simulink model "BCM_C1A_CombiSwitch_9"  (Simulink 9.2)
settings: Solver=FixedStepDiscrete  StartTime=0.0  StopTime=10.0  FixedStep=0.01  RelTol=1e-3
undefined symbols (not defined in the file or in its folder): TYP_VEHICLE_STATE
libraries: Renault_Library x8, library_BCM x1
settings Model: Creator=a205328  LastModifiedBy=40005501
settings DataIOCC: SaveFormat=StructureWithTime
settings OptimizationCC: ExpressionDepthLimit=2147483647
settings DebuggingCC: SolverPrmCheckMsg=warning  InheritedTsInSrcMsg=none
settings HardwareCC: TargetBitPerPointer=64  TargetBitPerSizeT=64  TargetBitPerPtrDiffT=64  TargetLongLongMode=on  TargetIntDivRoundTo=Zero  TargetEndianess=LittleEndian  TargetWordSize=64  TargetHWDeviceType=MATLAB Host  ProdEqTarget=off
settings GRTTargetCC: MatFileLogging=off  SupportNonFinite=off
settings ConfigComp: CovMetricSettings=dcmw  CovHTMLOptions=-sRT=1 -aTS=1 -bRG=1 -bTC=1 -hTR=0 -nFC=0 -scm=1 -bcm=1 -xEv=0  DVMaxTestCaseSteps=500  DVTestSuiteOptimization=CombinedObjectives (Nonlinear Extended)  DVDetectDeadLogic=on  DVDetectActiveLogic=on  DVDetectDivisionByZero=off  DVDetectIntegerOverflow=off

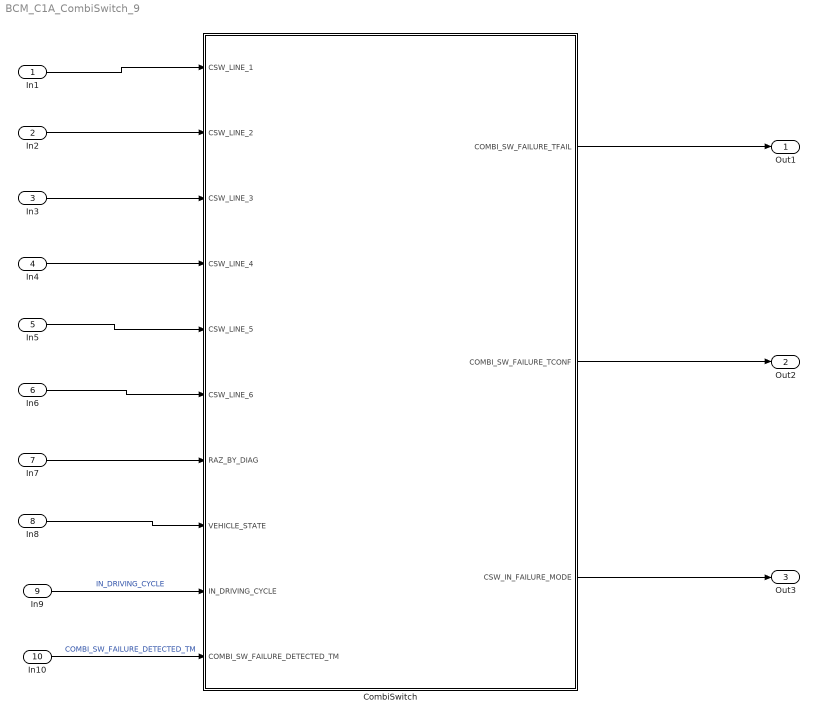
== system BCM_C1A_CombiSwitch_9 ==
  In1 : Inport
  In2 : Inport  Port=2
  In3 : Inport  Port=3
  In4 : Inport  Port=4
  In5 : Inport  Port=5
  In6 : Inport  Port=6
  In7 : Inport  Port=7
  In8 : Inport  Port=8
  In9 : Inport  Port=9
  In10 : Inport  Port=10
  CombiSwitch : Subsystem  Tag=[RUNNABLE]
  Out1 : Outport
  Out2 : Outport  Port=2
  Out3 : Outport  Port=3
  wires:
  In2/1 -> CombiSwitch/2(CSW_LINE_2)
  In3/1 -> CombiSwitch/3(CSW_LINE_3)
  In4/1 -> CombiSwitch/4(CSW_LINE_4)
  In7/1 -> CombiSwitch/7(RAZ_BY_DIAG)
  In1/1 -> CombiSwitch/1(CSW_LINE_1)
  In5/1 -> CombiSwitch/5(CSW_LINE_5)
  In6/1 -> CombiSwitch/6(CSW_LINE_6)
  In8/1 -> CombiSwitch/8(VEHICLE_STATE)
  CombiSwitch/1(COMBI_SW_FAILURE_TFAIL) -> Out1/1
  CombiSwitch/2(COMBI_SW_FAILURE_TCONF) -> Out2/1
  CombiSwitch/3(CSW_IN_FAILURE_MODE) -> Out3/1
  In9/1 -> CombiSwitch/9(IN_DRIVING_CYCLE)  "IN_DRIVING_CYCLE"
  In10/1 -> CombiSwitch/10(COMBI_SW_FAILURE_DETECTED_TM)  "COMBI_SW_FAILURE_DETECTED_TM"

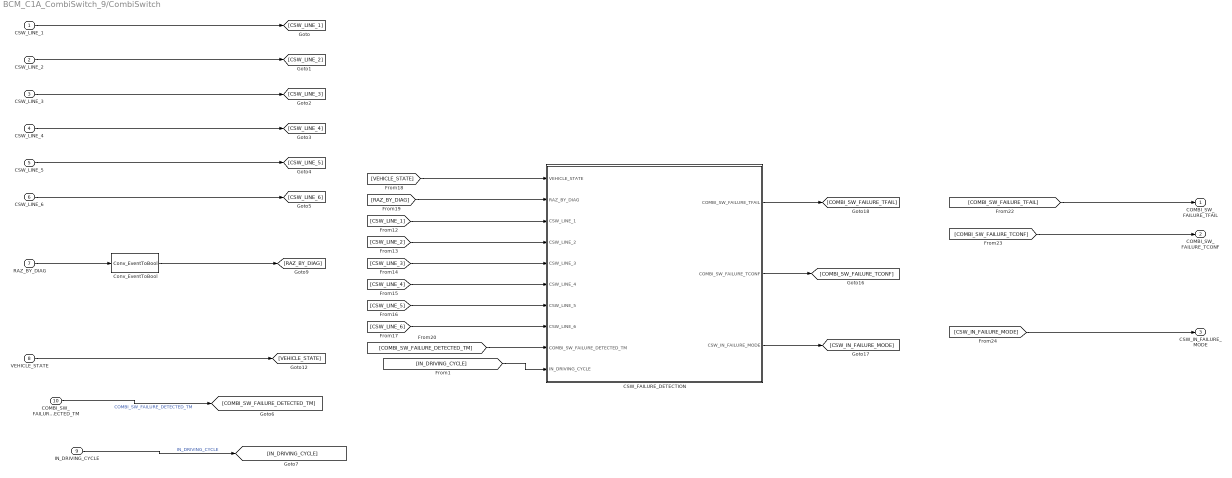
== system BCM_C1A_CombiSwitch_9/CombiSwitch ==
  CSW_LINE_1 : Inport  OutDataTypeStr=boolean  PortDimensions=6
      settings: AttributesFormatString=Type : %<OutDataTypeStr>
  CSW_LINE_2 : Inport  Port=2  OutDataTypeStr=boolean  PortDimensions=6
      settings: AttributesFormatString=Type : %<OutDataTypeStr>
  CSW_LINE_3 : Inport  Port=3  OutDataTypeStr=boolean  PortDimensions=6
      settings: AttributesFormatString=Type : %<OutDataTypeStr>
  CSW_LINE_4 : Inport  Port=4  OutDataTypeStr=boolean  PortDimensions=6
      settings: AttributesFormatString=Type : %<OutDataTypeStr>
  CSW_LINE_5 : Inport  Port=5  OutDataTypeStr=boolean  PortDimensions=6
      settings: AttributesFormatString=Type : %<OutDataTypeStr>
  CSW_LINE_6 : Inport  Port=6  OutDataTypeStr=boolean  PortDimensions=6
      settings: AttributesFormatString=Type : %<OutDataTypeStr>
  RAZ_BY_DIAG : Inport  Port=7  OutDataTypeStr=Enum: TYP_EVENT
      settings: AttributesFormatString=Type : %<OutDataTypeStr>
  VEHICLE_STATE : Inport  Port=8  OutDataTypeStr=Enum: TYP_VEHICLE_STATE
      settings: AttributesFormatString=Type : %<OutDataTypeStr>
  IN_DRIVING_CYCLE : Inport  Port=9  OutDataTypeStr=boolean
      settings: AttributesFormatString=Type : %<OutDataTypeStr>
  COMBI_SW_FAILURE_DETECTED_TM : Inport  Port=10  OutDataTypeStr=uint16
      settings: AttributesFormatString=Type : %<OutDataTypeStr>
  CSW_FAILURE_DETECTION : Subsystem  Description=|
      | RQT_BCM_CSV_1_1  
      | RQT_BCM_CSV_1_2  
      | RQT_BCM_CSV_1_3  
      | RQT_BCM_CSV_1_3_2
  Conv_EventToBool : library_BCM/Modeling/Conv_EventToBool
  COMBI_SW_FAILURE_TFAIL : Outport  OutDataTypeStr=boolean
      settings: AttributesFormatString=Type : %<OutDataTypeStr>\nInit :%<InitialOutput>
  COMBI_SW_FAILURE_TCONF : Outport  Port=2  OutDataTypeStr=boolean
      settings: AttributesFormatString=Type : %<OutDataTypeStr>\nInit :%<InitialOutput>
  CSW_IN_FAILURE_MODE : Outport  Port=3  OutDataTypeStr=boolean
      settings: AttributesFormatString=Type : %<OutDataTypeStr>\nInit :%<InitialOutput>
  wires:
  Conv_EventToBool/1 -> [RAZ_BY_DIAG]
  [COMBI_SW_FAILURE_DETECTED_TM] -> CSW_FAILURE_DETECTION/9(COMBI_SW_FAILURE_DETECTED_TM)
  [CSW_LINE_6] -> CSW_FAILURE_DETECTION/8(CSW_LINE_6)
  [CSW_LINE_5] -> CSW_FAILURE_DETECTION/7(CSW_LINE_5)
  [CSW_LINE_4] -> CSW_FAILURE_DETECTION/6(CSW_LINE_4)
  [CSW_LINE_3] -> CSW_FAILURE_DETECTION/5(CSW_LINE_3)
  [CSW_LINE_2] -> CSW_FAILURE_DETECTION/4(CSW_LINE_2)
  [CSW_LINE_1] -> CSW_FAILURE_DETECTION/3(CSW_LINE_1)
  [RAZ_BY_DIAG] -> CSW_FAILURE_DETECTION/2(RAZ_BY_DIAG)
  [VEHICLE_STATE] -> CSW_FAILURE_DETECTION/1(VEHICLE_STATE)
  CSW_LINE_6/1 -> [CSW_LINE_6]
  CSW_LINE_5/1 -> [CSW_LINE_5]
  CSW_LINE_4/1 -> [CSW_LINE_4]
  CSW_LINE_3/1 -> [CSW_LINE_3]
  CSW_LINE_2/1 -> [CSW_LINE_2]
  CSW_LINE_1/1 -> [CSW_LINE_1]
  RAZ_BY_DIAG/1 -> Conv_EventToBool/1
  VEHICLE_STATE/1 -> [VEHICLE_STATE]
  CSW_FAILURE_DETECTION/2(COMBI_SW_FAILURE_TCONF) -> [COMBI_SW_FAILURE_TCONF]
  CSW_FAILURE_DETECTION/3(CSW_IN_FAILURE_MODE) -> [CSW_IN_FAILURE_MODE]
  CSW_FAILURE_DETECTION/1(COMBI_SW_FAILURE_TFAIL) -> [COMBI_SW_FAILURE_TFAIL]
  [COMBI_SW_FAILURE_TFAIL] -> COMBI_SW_FAILURE_TFAIL/1
  [COMBI_SW_FAILURE_TCONF] -> COMBI_SW_FAILURE_TCONF/1
  [CSW_IN_FAILURE_MODE] -> CSW_IN_FAILURE_MODE/1
  [IN_DRIVING_CYCLE] -> CSW_FAILURE_DETECTION/10(IN_DRIVING_CYCLE)
  IN_DRIVING_CYCLE/1 -> [IN_DRIVING_CYCLE]  "IN_DRIVING_CYCLE"
  COMBI_SW_FAILURE_DETECTED_TM/1 -> [COMBI_SW_FAILURE_DETECTED_TM]  "COMBI_SW_FAILURE_DETECTED_TM"

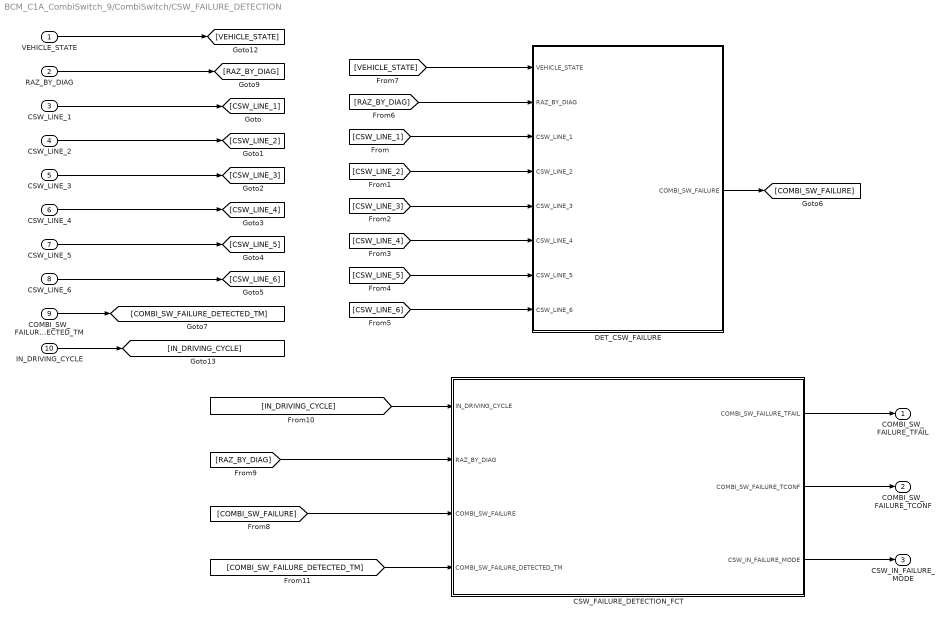
== system BCM_C1A_CombiSwitch_9/CombiSwitch/CSW_FAILURE_DETECTION ==
  VEHICLE_STATE : Inport  OutDataTypeStr=Enum: TYP_VEHICLE_STATE
      settings: AttributesFormatString=Type : %<OutDataTypeStr>
  RAZ_BY_DIAG : Inport  Port=2  OutDataTypeStr=boolean
      settings: AttributesFormatString=Type : %<OutDataTypeStr>
  CSW_LINE_1 : Inport  Port=3  OutDataTypeStr=boolean  PortDimensions=6
      settings: AttributesFormatString=Type : %<OutDataTypeStr>
  CSW_LINE_2 : Inport  Port=4  OutDataTypeStr=boolean  PortDimensions=6
      settings: AttributesFormatString=Type : %<OutDataTypeStr>
  CSW_LINE_3 : Inport  Port=5  OutDataTypeStr=boolean  PortDimensions=6
      settings: AttributesFormatString=Type : %<OutDataTypeStr>
  CSW_LINE_4 : Inport  Port=6  OutDataTypeStr=boolean  PortDimensions=6
      settings: AttributesFormatString=Type : %<OutDataTypeStr>
  CSW_LINE_5 : Inport  Port=7  OutDataTypeStr=boolean  PortDimensions=6
      settings: AttributesFormatString=Type : %<OutDataTypeStr>
  CSW_LINE_6 : Inport  Port=8  OutDataTypeStr=boolean  PortDimensions=6
      settings: AttributesFormatString=Type : %<OutDataTypeStr>
  COMBI_SW_FAILURE_DETECTED_TM : Inport  Port=9  OutDataTypeStr=uint16
      settings: AttributesFormatString=Type : %<OutDataTypeStr>
  IN_DRIVING_CYCLE : Inport  Port=10  OutDataTypeStr=boolean
      settings: AttributesFormatString=Type : %<OutDataTypeStr>
  CSW_FAILURE_DETECTION_FCT : Stateflow chart  Description=RQT_BCM_CSV_1_0_1  TreatAsAtomicUnit=on
  DET_CSW_FAILURE : Subsystem
  COMBI_SW_FAILURE_TFAIL : Outport  OutDataTypeStr=boolean
      settings: AttributesFormatString=Type : %<OutDataTypeStr>\nInit :%<InitialOutput>
  COMBI_SW_FAILURE_TCONF : Outport  Port=2  OutDataTypeStr=boolean
      settings: AttributesFormatString=Type : %<OutDataTypeStr>\nInit :%<InitialOutput>
  CSW_IN_FAILURE_MODE : Outport  Port=3  OutDataTypeStr=boolean
      settings: AttributesFormatString=Type : %<OutDataTypeStr>\nInit :%<InitialOutput>
  wires:
  IN_DRIVING_CYCLE/1 -> [IN_DRIVING_CYCLE]
  CSW_FAILURE_DETECTION_FCT/2(COMBI_SW_FAILURE_TCONF) -> COMBI_SW_FAILURE_TCONF/1
  [COMBI_SW_FAILURE_DETECTED_TM] -> CSW_FAILURE_DETECTION_FCT/4(COMBI_SW_FAILURE_DETECTED_TM)
  [RAZ_BY_DIAG] -> CSW_FAILURE_DETECTION_FCT/2(RAZ_BY_DIAG)
  [IN_DRIVING_CYCLE] -> CSW_FAILURE_DETECTION_FCT/1(IN_DRIVING_CYCLE)
  [COMBI_SW_FAILURE] -> CSW_FAILURE_DETECTION_FCT/3(COMBI_SW_FAILURE)
  COMBI_SW_FAILURE_DETECTED_TM/1 -> [COMBI_SW_FAILURE_DETECTED_TM]
  [CSW_LINE_6] -> DET_CSW_FAILURE/8(CSW_LINE_6)
  [CSW_LINE_5] -> DET_CSW_FAILURE/7(CSW_LINE_5)
  [CSW_LINE_4] -> DET_CSW_FAILURE/6(CSW_LINE_4)
  [CSW_LINE_3] -> DET_CSW_FAILURE/5(CSW_LINE_3)
  [CSW_LINE_2] -> DET_CSW_FAILURE/4(CSW_LINE_2)
  [CSW_LINE_1] -> DET_CSW_FAILURE/3(CSW_LINE_1)
  [RAZ_BY_DIAG] -> DET_CSW_FAILURE/2(RAZ_BY_DIAG)
  [VEHICLE_STATE] -> DET_CSW_FAILURE/1(VEHICLE_STATE)
  CSW_LINE_6/1 -> [CSW_LINE_6]
  CSW_LINE_5/1 -> [CSW_LINE_5]
  CSW_LINE_4/1 -> [CSW_LINE_4]
  CSW_LINE_3/1 -> [CSW_LINE_3]
  CSW_LINE_2/1 -> [CSW_LINE_2]
  CSW_LINE_1/1 -> [CSW_LINE_1]
  RAZ_BY_DIAG/1 -> [RAZ_BY_DIAG]
  VEHICLE_STATE/1 -> [VEHICLE_STATE]
  CSW_FAILURE_DETECTION_FCT/3(CSW_IN_FAILURE_MODE) -> CSW_IN_FAILURE_MODE/1
  CSW_FAILURE_DETECTION_FCT/1(COMBI_SW_FAILURE_TFAIL) -> COMBI_SW_FAILURE_TFAIL/1
  DET_CSW_FAILURE/1(COMBI_SW_FAILURE) -> [COMBI_SW_FAILURE]

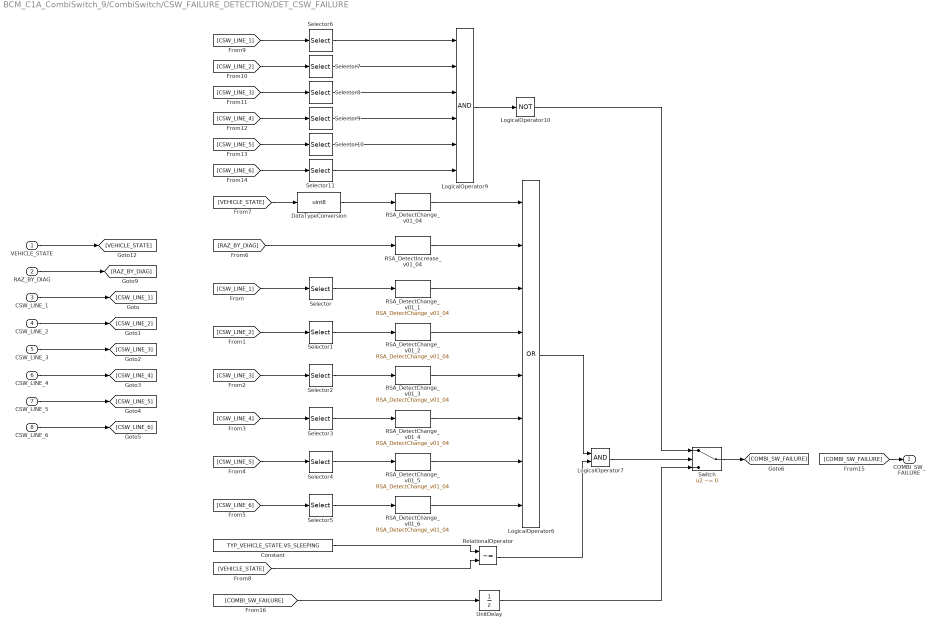
== system BCM_C1A_CombiSwitch_9/CombiSwitch/CSW_FAILURE_DETECTION/DET_CSW_FAILURE ==
  VEHICLE_STATE : Inport  OutDataTypeStr=Enum: TYP_VEHICLE_STATE
      settings: AttributesFormatString=Type : %<OutDataTypeStr>
  RAZ_BY_DIAG : Inport  Port=2  OutDataTypeStr=boolean
      settings: AttributesFormatString=Type : %<OutDataTypeStr>
  CSW_LINE_1 : Inport  Port=3  OutDataTypeStr=boolean  PortDimensions=6
      settings: AttributesFormatString=Type : %<OutDataTypeStr>
  CSW_LINE_2 : Inport  Port=4  OutDataTypeStr=boolean  PortDimensions=6
      settings: AttributesFormatString=Type : %<OutDataTypeStr>
  CSW_LINE_3 : Inport  Port=5  OutDataTypeStr=boolean  PortDimensions=6
      settings: AttributesFormatString=Type : %<OutDataTypeStr>
  CSW_LINE_4 : Inport  Port=6  OutDataTypeStr=boolean  PortDimensions=6
      settings: AttributesFormatString=Type : %<OutDataTypeStr>
  CSW_LINE_5 : Inport  Port=7  OutDataTypeStr=boolean  PortDimensions=6
      settings: AttributesFormatString=Type : %<OutDataTypeStr>
  CSW_LINE_6 : Inport  Port=8  OutDataTypeStr=boolean  PortDimensions=6
      settings: AttributesFormatString=Type : %<OutDataTypeStr>
  Constant : Constant  Value=TYP_VEHICLE_STATE.VS_SLEEPING  OutDataTypeStr=Enum: TYP_VEHICLE_STATE  SampleTime=-1
  DataTypeConversion : DataTypeConversion  OutDataTypeStr=uint8  RndMeth=Zero
      settings: AttributesFormatString=Saturation:%<SaturateOnIntegerOverflow>
  LogicalOperator10 : Logic  Operator=NOT  Inputs=1  OutDataTypeStr=boolean
  LogicalOperator6 : Logic  Operator=OR  Inputs=8  OutDataTypeStr=boolean
  LogicalOperator7 : Logic  OutDataTypeStr=boolean
  LogicalOperator9 : Logic  Inputs=6  OutDataTypeStr=boolean
  RSA_DetectChange_v01_04 : Renault_Library/Complex blocks/Logic & Bit Operations/RSA_DetectChange_v01_04  Tag=[LIB]  chkini=on  vinit=false
      settings: AttributesFormatString=%<MaskType> : Ver : 01.04\nCompare the Input with Initial Value = %<chkini>\nInitial Value : = %<vinit>
  RSA_DetectChange_v01_{1..6} (6 alike) : Renault_Library/Complex blocks/Logic & Bit Operations/RSA_DetectChange_v01_04  Tag=[LIB]  chkini=on  vinit=false
      settings: AttributesFormatString=%<MaskType> : Ver : 01.04\nCompare the Input with Initial Value = %<chkini>\nInitial Value : = %<vinit>
  RSA_DetectIncrease_v01_04 : Renault_Library/Complex blocks/Logic & Bit Operations/RSA_DetectIncrease_v01_04  Tag=[LIB]  chkini=on  vinit=false
      settings: AttributesFormatString=%<MaskType> : Ver : 01.04\nCompare the Input with Initial Value = %<chkini>\nInitial Value : = %<vinit>
  RelationalOperator : RelationalOperator  Operator=~=  OutDataTypeStr=boolean  RndMeth=Nearest  InputSameDT=on
  Selector : Selector  IndexMode=Zero-based  InputPortWidth=6  IndexOptions=Index vector (dialog)  Indices=[0]  OutputSizes=1
  Selector1 : Selector  IndexMode=Zero-based  InputPortWidth=6  IndexOptions=Index vector (dialog)  Indices=[1]  OutputSizes=1
  Selector10 : Selector  IndexMode=Zero-based  InputPortWidth=6  IndexOptions=Index vector (dialog)  Indices=[4]  OutputSizes=1
  Selector11 : Selector  IndexMode=Zero-based  InputPortWidth=6  IndexOptions=Index vector (dialog)  Indices=[5]  OutputSizes=1
  Selector2 : Selector  IndexMode=Zero-based  InputPortWidth=6  IndexOptions=Index vector (dialog)  Indices=[2]  OutputSizes=1
  Selector3 : Selector  IndexMode=Zero-based  InputPortWidth=6  IndexOptions=Index vector (dialog)  Indices=[3]  OutputSizes=1
  Selector4 : Selector  IndexMode=Zero-based  InputPortWidth=6  IndexOptions=Index vector (dialog)  Indices=[4]  OutputSizes=1
  Selector5 : Selector  IndexMode=Zero-based  InputPortWidth=6  IndexOptions=Index vector (dialog)  Indices=[5]  OutputSizes=1
  Selector6 : Selector  IndexMode=Zero-based  InputPortWidth=6  IndexOptions=Index vector (dialog)  Indices=[0]  OutputSizes=1
  Selector7 : Selector  IndexMode=Zero-based  InputPortWidth=6  IndexOptions=Index vector (dialog)  Indices=[1]  OutputSizes=1
  Selector8 : Selector  IndexMode=Zero-based  InputPortWidth=6  IndexOptions=Index vector (dialog)  Indices=[2]  OutputSizes=1
  Selector9 : Selector  IndexMode=Zero-based  InputPortWidth=6  IndexOptions=Index vector (dialog)  Indices=[3]  OutputSizes=1
  Switch : Switch  Criteria=u2 ~= 0  RndMeth=Zero  InputSameDT=on
      settings: AttributesFormatString=Criteria=%<Criteria>
  UnitDelay : UnitDelay  InitialCondition=false  SampleTime=-1
      settings: AttributesFormatString=IC = %<X0>
  COMBI_SW_FAILURE : Outport  OutDataTypeStr=boolean
      settings: AttributesFormatString=Type : %<OutDataTypeStr>\nInit :%<InitialOutput>
  wires:
  LogicalOperator9/1 -> LogicalOperator10/1
  Selector6/1 -> LogicalOperator9/1
  Selector8/1 -> LogicalOperator9/3
  Selector9/1 -> LogicalOperator9/4
  Selector10/1 -> LogicalOperator9/5
  Selector11/1 -> LogicalOperator9/6
  Selector7/1 -> LogicalOperator9/2
  [CSW_LINE_6] -> Selector11/1
  [CSW_LINE_5] -> Selector10/1
  [CSW_LINE_4] -> Selector9/1
  [CSW_LINE_3] -> Selector8/1
  [CSW_LINE_2] -> Selector7/1
  [CSW_LINE_1] -> Selector6/1
  LogicalOperator6/1 -> LogicalOperator7/1
  RelationalOperator/1 -> LogicalOperator7/2
  [VEHICLE_STATE] -> RelationalOperator/2
  Constant/1 -> RelationalOperator/1
  [RAZ_BY_DIAG] -> RSA_DetectIncrease_v01_04/1
  DataTypeConversion/1 -> RSA_DetectChange_v01_04/1
  [VEHICLE_STATE] -> DataTypeConversion/1
  Selector2/1 -> RSA_DetectChange_v01_3/1
  Selector3/1 -> RSA_DetectChange_v01_4/1
  Selector4/1 -> RSA_DetectChange_v01_5/1
  Selector5/1 -> RSA_DetectChange_v01_6/1
  Selector1/1 -> RSA_DetectChange_v01_2/1
  Selector/1 -> RSA_DetectChange_v01_1/1
  [CSW_LINE_6] -> Selector5/1
  [CSW_LINE_5] -> Selector4/1
  [CSW_LINE_4] -> Selector3/1
  [CSW_LINE_3] -> Selector2/1
  [CSW_LINE_2] -> Selector1/1
  [CSW_LINE_1] -> Selector/1
  CSW_LINE_6/1 -> [CSW_LINE_6]
  CSW_LINE_5/1 -> [CSW_LINE_5]
  CSW_LINE_4/1 -> [CSW_LINE_4]
  CSW_LINE_3/1 -> [CSW_LINE_3]
  CSW_LINE_2/1 -> [CSW_LINE_2]
  CSW_LINE_1/1 -> [CSW_LINE_1]
  RAZ_BY_DIAG/1 -> [RAZ_BY_DIAG]
  VEHICLE_STATE/1 -> [VEHICLE_STATE]
  LogicalOperator7/1 -> Switch/2
  LogicalOperator10/1 -> Switch/1
  Switch/1 -> [COMBI_SW_FAILURE]
  [COMBI_SW_FAILURE] -> UnitDelay/1
  [COMBI_SW_FAILURE] -> COMBI_SW_FAILURE/1
  UnitDelay/1 -> Switch/3
  RSA_DetectChange_v01_6/1 -> LogicalOperator6/8
  RSA_DetectChange_v01_5/1 -> LogicalOperator6/7
  RSA_DetectChange_v01_4/1 -> LogicalOperator6/6
  RSA_DetectChange_v01_3/1 -> LogicalOperator6/5
  RSA_DetectChange_v01_2/1 -> LogicalOperator6/4
  RSA_DetectChange_v01_1/1 -> LogicalOperator6/3
  RSA_DetectIncrease_v01_04/1 -> LogicalOperator6/2
  RSA_DetectChange_v01_04/1 -> LogicalOperator6/1

== stateflow chart CombiSwitch/CSW_FAILURE_DETECTION/CSW_FAILURE_DETECTION_FCT ==
  state CSW_FAILURE_DETECTION
    state NO_CSW_FAILURE_DETECTION_TEST
    state CSW_FAILURE_DETECTION_TEST
      state CSW_FAILURE_CONFIRMATION
        entry:
        COMBI_SW_FAILURE_TFAIL=true;
        COMBI_SW_FAILURE_TCONF=true;
        CSW_IN_FAILURE_MODE=true;
      state NO_CSW_FAILURE_CONFIRMATION
        state NO_CSW_FAILURE
          entry:
          COMBI_SW_FAILURE_TFAIL=false;
          COMBI_SW_FAILURE_TCONF=false;
          CSW_IN_FAILURE_MODE=false;
        state WAITING_CSW_FAILURE_CONFIRMATION
          entry:
          COMBI_SW_FAILURE_TFAIL=true;
        state WAITING_CSW_FAILURE_COME_BACK_IN_NORMAL
        (default) -> NO_CSW_FAILURE
        NO_CSW_FAILURE -> WAITING_CSW_FAILURE_CONFIRMATION : [COMBI_SW_FAILURE]
        WAITING_CSW_FAILURE_CONFIRMATION -> NO_CSW_FAILURE [order 1] : [!COMBI_SW_FAILURE ...
            | && !COMBI_SW_FAILURE_TCONF]
        WAITING_CSW_FAILURE_COME_BACK_IN_NORMAL -> NO_CSW_FAILURE [order 2] : after(COMBI_SW_FAILURE_DETECTED_TM,tick)
        WAITING_CSW_FAILURE_COME_BACK_IN_NORMAL -> WAITING_CSW_FAILURE_CONFIRMATION [order 1] : [COMBI_SW_FAILURE]
        WAITING_CSW_FAILURE_CONFIRMATION -> WAITING_CSW_FAILURE_COME_BACK_IN_NORMAL [order 2] : [!COMBI_SW_FAILURE ...
            | && COMBI_SW_FAILURE_TCONF]
      (junction 11) -> NO_CSW_FAILURE_CONFIRMATION [order 2]
      CSW_FAILURE_CONFIRMATION -> WAITING_CSW_FAILURE_COME_BACK_IN_NORMAL : [!COMBI_SW_FAILURE]
      (default) -> (junction 11)
      (junction 11) -> CSW_FAILURE_CONFIRMATION [order 1] : [COMBI_SW_FAILURE_TCONF==true ...
          | && COMBI_SW_FAILURE==true]
      WAITING_CSW_FAILURE_CONFIRMATION -> CSW_FAILURE_CONFIRMATION [order 3] : after(COMBI_SW_FAILURE_DETECTED_TM,tick)
    (junction 17) -> NO_CSW_FAILURE_DETECTION_TEST [order 2]
    NO_CSW_FAILURE_DETECTION_TEST -> CSW_FAILURE_DETECTION_TEST : [IN_DRIVING_CYCLE]
    CSW_FAILURE_DETECTION_TEST -> NO_CSW_FAILURE_DETECTION_TEST : [!IN_DRIVING_CYCLE]
    (default) -> (junction 17)
    (junction 17) -> CSW_FAILURE_DETECTION_TEST [order 1] : [IN_DRIVING_CYCLE]
  (default) -> CSW_FAILURE_DETECTION : {
      | COMBI_SW_FAILURE_TFAIL=false;
      | COMBI_SW_FAILURE_TCONF=false;
      | CSW_IN_FAILURE_MODE=false;
      | }
  CSW_FAILURE_DETECTION -> CSW_FAILURE_DETECTION : [hasChangedFrom(RAZ_BY_DIAG,true)]
      | {
      | COMBI_SW_FAILURE_TFAIL=false;
      | COMBI_SW_FAILURE_TCONF=false;
      | CSW_IN_FAILURE_MODE=false;
      | }
  data: COMBI_SW_FAILURE_TFAIL output boolean; IN_DRIVING_CYCLE input boolean; RAZ_BY_DIAG input boolean; COMBI_SW_FAILURE input boolean; COMBI_SW_FAILURE_DETECTED_TM input uint16; COMBI_SW_FAILURE_TCONF output boolean; CSW_IN_FAILURE_MODE output boolean
